simulink model "two_tanks"  (R2018b)
settings: Solver=FixedStepAuto  StartTime=0.0  StopTime=60  FixedStep=0.1  RelTol=1e-3
model workspace (MATLAB code in the model file):
  | A1 = 1;
  | a1 = 0.1*0.1;
  | A2 = A1;
  | a2 = a1;
  | h10 = 1;
  | h20=1;
libraries: simulink x1
settings Model: EnablePacing=on  Creator=kjartan  LastModifiedBy=kjartan

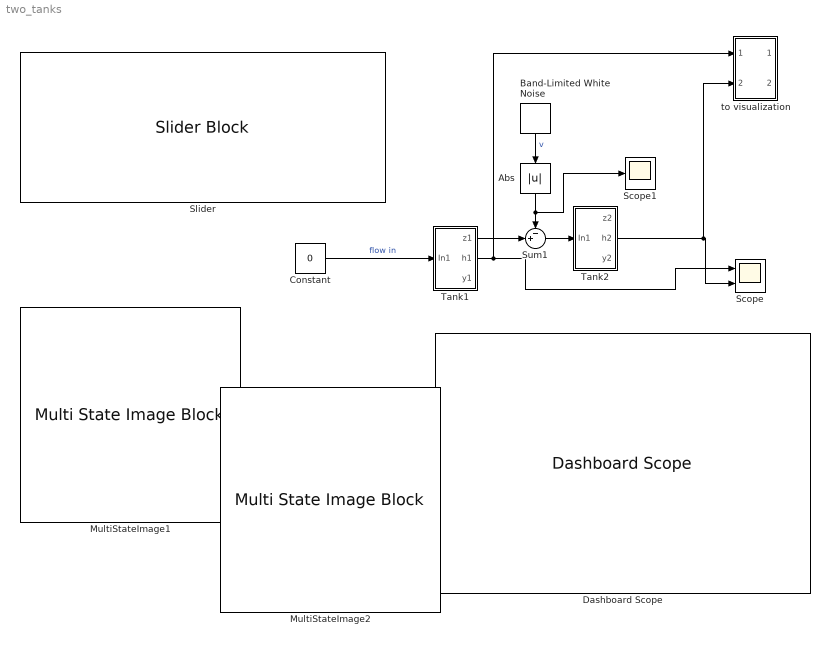
== system two_tanks ==
  Abs : Abs
  Band-Limited White Noise : simulink/Sources/Band-Limited White Noise  Cov=0.01*0.01  Ts=3  seed=[23341]
  Constant : Constant  Value=0
  Dashboard Scope : DashboardScope  WebBlockId=50  Ymin=0  Ymax=2
  MultiStateImage1 : MultiStateImageBlock  WebBlockId=71
  MultiStateImage2 : MultiStateImageBlock  WebBlockId=74
  Scope : Scope  NumInputPorts=2
  Scope1 : Scope
  Slider : SliderBlock  WebBlockId=45  ScaleMax=0.10000000000000001
  Sum1 : Sum  Inputs=-+|
  Tank1 : Subsystem
  Tank2 : Subsystem
  to visualization : Subsystem
  wires:
  Constant/1 -> Tank1/1(In1)  "flow in"
  Tank1/1(z1) -> Sum1/2
  Tank1/2(h1) -> to visualization/1(In2), Scope/1
  Tank2/2(h2) -> to visualization/2(In1), Scope/2
  Sum1/1 -> Tank2/1(In1)
  Band-Limited White Noise/1 -> Abs/1  "v"
  Abs/1 -> Scope1/1, Sum1/1

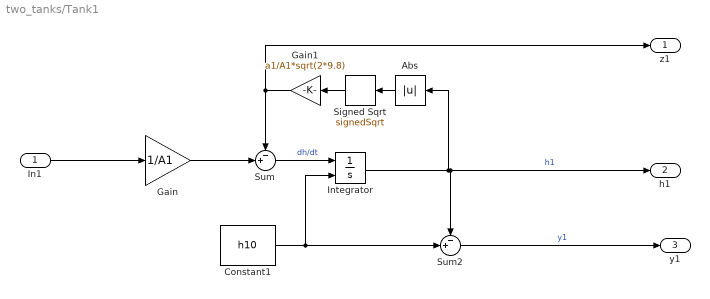
== system two_tanks/Tank1 ==
  In1 : Inport
  Abs : Abs
  Constant1 : Constant  Value=h10
  Gain : Gain  Gain=1/A1
  Gain1 : Gain  Gain=a1/A1*sqrt(2*9.8)
  Integrator : Integrator  InitialConditionSource=external  InitialCondition=h10
  Signed Sqrt : Sqrt  Operator=signedSqrt  SaturateOnIntegerOverflow=on
  Sum : Sum  Inputs=-+|
  Sum2 : Sum  Inputs=-+|
  z1 : Outport
  h1 : Outport  Port=2
  y1 : Outport  Port=3
  wires:
  Gain1/1 -> z1/1, Sum/1
  Gain/1 -> Sum/2
  Sum/1 -> Integrator/1  "dh/dt"
  In1/1 -> Gain/1
  Sum2/1 -> y1/1  "y1"
  Signed Sqrt/1 -> Gain1/1
  Integrator/1 -> h1/1, Sum2/1, Abs/1  "h1"
  Abs/1 -> Signed Sqrt/1
  Constant1/1 -> Sum2/2, Integrator/2

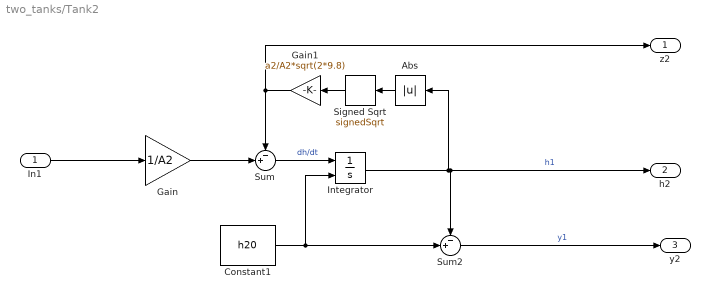
== system two_tanks/Tank2 ==
  In1 : Inport
  Abs : Abs
  Constant1 : Constant  Value=h20
  Gain : Gain  Gain=1/A2
  Gain1 : Gain  Gain=a2/A2*sqrt(2*9.8)
  Integrator : Integrator  InitialConditionSource=external  InitialCondition=h10
  Signed Sqrt : Sqrt  Operator=signedSqrt  SaturateOnIntegerOverflow=on
  Sum : Sum  Inputs=-+|
  Sum2 : Sum  Inputs=-+|
  z2 : Outport
  h2 : Outport  Port=2
  y2 : Outport  Port=3
  wires:
  Gain1/1 -> z2/1, Sum/1
  Gain/1 -> Sum/2
  Sum/1 -> Integrator/1  "dh/dt"
  In1/1 -> Gain/1
  Sum2/1 -> y2/1  "y1"
  Signed Sqrt/1 -> Gain1/1
  Integrator/1 -> h2/1, Sum2/1, Abs/1  "h1"
  Abs/1 -> Signed Sqrt/1
  Constant1/1 -> Sum2/2, Integrator/2

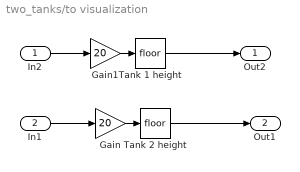
== system two_tanks/to visualization ==
  In2 : Inport
  In1 : Inport  Port=2
  Gain : Gain  Gain=20
  Gain1 : Gain  Gain=20
  Tank 1 height : Rounding
  Tank 2 height : Rounding
  Out2 : Outport
  Out1 : Outport  Port=2
  wires:
  Tank 2 height/1 -> Out1/1
  Gain/1 -> Tank 2 height/1
  In1/1 -> Gain/1
  Tank 1 height/1 -> Out2/1
  Gain1/1 -> Tank 1 height/1
  In2/1 -> Gain1/1
